simulink model "pos_pid_mbd_sl"  (Simulink 7.9)
settings: Solver=FixedStepDiscrete  StartTime=0.0  StopTime=tfinal  FixedStep=ts  RelTol=1e-3
values from neighbouring files (symbols this model uses):
  denpd = [1 -1.93941306281 0.939413062813]    [model_data.mat]
  dist = 0    [pos_pd_mbd.m]    (also in pos_pid2_mbd.m; pos_pid_mbd.m = 2; pos_pid_set.m; pos_tdof_mbd.m)
  Kd = -((p1+p2+p3)*T + 1)/K    [ipd_ff.m]    (also in pid_compare.m; pos_id_verify.m = 0; pos_pd_mbd.m = -((p1+p2)*T + 1)/K; pos_pid2_mbd.m)
  Ki = -p1*p2*p3*T/K    [ipd_ff.m]    (also in pid_compare.m; pos_id_verify.m = 0; pos_pd_mbd.m = 0; pos_pid2_mbd.m)
  Kp = (p1*p2 + p2*p3 + p3*p1)*T/K    [ipd_ff.m]    (also in pid_compare.m; pos_id_verify.m = Kp_id; pos_pd_mbd.m = p1*p2*T/K; pos_pid2_mbd.m)
  numpd = [0 0.223445736614 0.218838904848]    [model_data.mat]
  r = 60    [pos_id_step.m]    (also in pos_pd_mbd.m; pos_pid2_mbd.m; pos_pid_mbd.m; pos_pid_set.m)
  r_cyc = 8    [pos_id_step.m]    (also in pos_pd_mbd.m = 4; pos_pid2_mbd.m = 4; pos_pid_mbd.m = 4; pos_pid_set.m = 4)
  ts = 1/50    (= 0.02)    [sim_init.m]    (also in sim_param.mat)
undefined symbols (not defined in the file or in its folder): DiscIntNeverNeededParam
libraries: arduino_io_lib x5, simulink x2
settings Model: Creator=hirata  LastModifiedBy=hirata
settings DebuggingCC: FcnCallInpInsideContextMsg=Use local settings
settings GRTTargetCC: CombineOutputUpdateFcns=off  GRTInterface=on

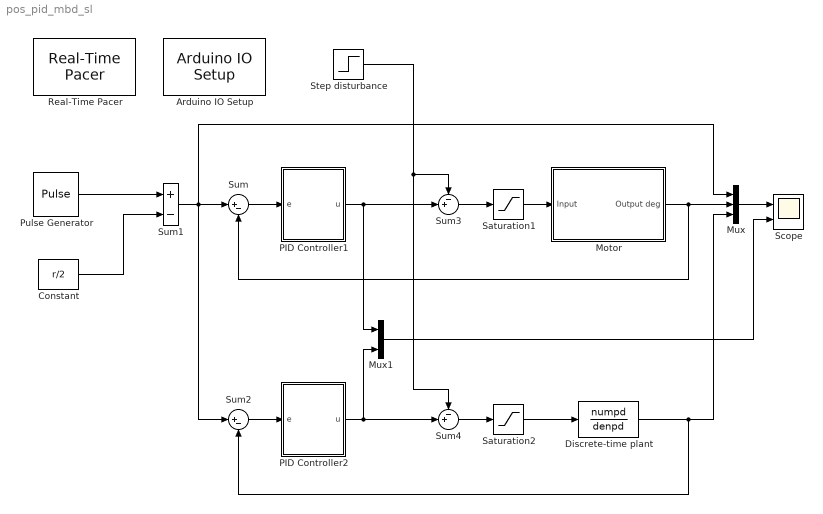
== system pos_pid_mbd_sl ==
  Arduino IO Setup : arduino_io_lib/Arduino IO Setup  Priority=3  arduinoVar=Temporary arduino variable: Arduino1  workspaceVarName=a  comPort=COM3
  Constant : Constant  Value=r/2
  Discrete-time plant : DiscreteTransferFcn  Numerator=numpd  Denominator=denpd
  Motor : Subsystem
  Mux : Mux  Inputs=3
  Mux1 : Mux  Inputs=2
  PID Controller1 : Subsystem
  PID Controller2 : Subsystem
  Pulse Generator : DiscretePulseGenerator  PulseType=Time based  Amplitude=r  Period=r_cyc  PulseWidth=50
  Real-Time Pacer : arduino_io_lib/Real-Time Pacer  simTimePerRealTime=1
  Saturation1 : Saturate  UpperLimit=5  LowerLimit=-5
  Saturation2 : Saturate  UpperLimit=5  LowerLimit=-5
  Scope : Scope  NumInputPorts=2
      settings: TimeRange=8  YMin=-80~-5  YMax=80~5  SaveName=yout
  Step disturbance : Step  Time=r_cyc/4  After=dist  SampleTime=ts
  Sum : Sum  Inputs=|+-
  Sum1 : Sum  Inputs=+-
  Sum2 : Sum  Inputs=|+-
  Sum3 : Sum  Inputs=-+|
  Sum4 : Sum  Inputs=-+|
  wires:
  PID Controller1/1(u) -> Mux1/1, Sum3/2
  Sum/1 -> PID Controller1/1(e)
  Sum1/1 -> Sum/1, Mux/1, Sum2/1
  Motor/1(Output deg) -> Sum/2, Mux/2
  Pulse Generator/1 -> Sum1/1
  Constant/1 -> Sum1/2
  Mux/1 -> Scope/1
  PID Controller2/1(u) -> Mux1/2, Sum4/2
  Sum2/1 -> PID Controller2/1(e)
  Mux1/1 -> Scope/2
  Discrete-time plant/1 -> Sum2/2, Mux/3
  Step disturbance/1 -> Sum4/1, Sum3/1
  Sum3/1 -> Saturation1/1
  Sum4/1 -> Saturation2/1
  Saturation1/1 -> Motor/1(Input)
  Saturation2/1 -> Discrete-time plant/1

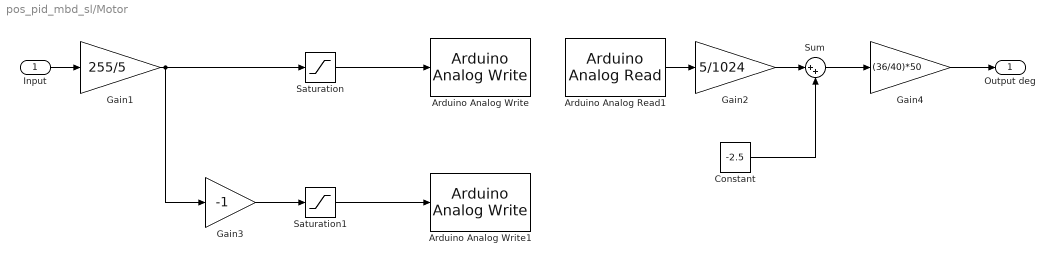
== system pos_pid_mbd_sl/Motor ==
  Input : Inport
  Arduino Analog Read1 : arduino_io_lib/Arduino Analog Read  arduinoVar=Temporary arduino variable: Arduino1  arduinoPin=0  T=ts
  Arduino Analog Write : arduino_io_lib/Arduino Analog Write  arduinoVar=Temporary arduino variable: Arduino1  arduinoPin=3  T=ts
  Arduino Analog Write1 : arduino_io_lib/Arduino Analog Write  arduinoVar=Temporary arduino variable: Arduino1  arduinoPin=5  T=ts
  Constant : Constant  Value=-2.5
  Gain1 : Gain  Gain=255/5
  Gain2 : Gain  Gain=5/1024
  Gain3 : Gain  Gain=-1
  Gain4 : Gain  Gain=(36/40)*50
  Saturation : Saturate  UpperLimit=255  LowerLimit=0
  Saturation1 : Saturate  UpperLimit=255  LowerLimit=0
  Sum : Sum  Inputs=|++
  Output deg : Outport
  wires:
  Input/1 -> Gain1/1
  Arduino Analog Read1/1 -> Gain2/1
  Saturation/1 -> Arduino Analog Write/1
  Gain1/1 -> Gain3/1, Saturation/1
  Saturation1/1 -> Arduino Analog Write1/1
  Gain4/1 -> Output deg/1
  Gain2/1 -> Sum/1
  Sum/1 -> Gain4/1
  Constant/1 -> Sum/2
  Gain3/1 -> Saturation1/1

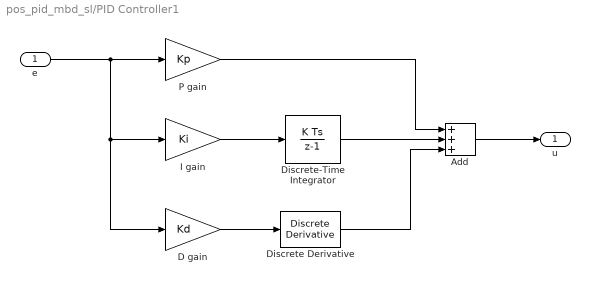
== system pos_pid_mbd_sl/PID Controller1 ==
  e : Inport
  Add : Sum  Inputs=+++
  D gain : Gain  Gain=Kd
  Discrete Derivative : simulink/Discrete/Discrete Derivative  gainval=1.0  ICPrevScaledInput=0.0  InputProcessing=Inherited  OutMin=[]  OutMax=[]  OutDataType=fixdt(1, 16)  OutScaling=2^-10  DoSatur=off
  Discrete-Time Integrator : DiscreteIntegrator  SampleTime=ts  ICPrevOutput=DiscIntNeverNeededParam  ICPrevScaledInput=DiscIntNeverNeededParam
  I gain : Gain  Gain=Ki
  P gain : Gain  Gain=Kp
  u : Outport
  wires:
  I gain/1 -> Discrete-Time Integrator/1
  P gain/1 -> Add/1
  Discrete-Time Integrator/1 -> Add/2
  e/1 -> P gain/1, I gain/1, D gain/1
  Add/1 -> u/1
  Discrete Derivative/1 -> Add/3
  D gain/1 -> Discrete Derivative/1

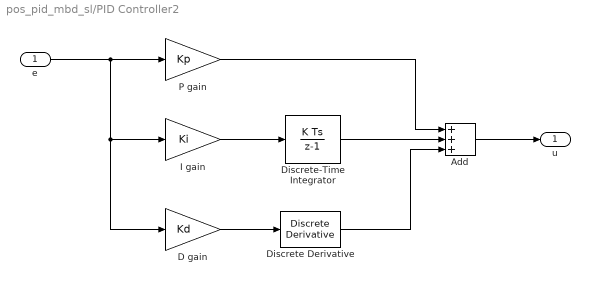
== system pos_pid_mbd_sl/PID Controller2 ==
  e : Inport
  Add : Sum  Inputs=+++
  D gain : Gain  Gain=Kd
  Discrete Derivative : simulink/Discrete/Discrete Derivative  gainval=1.0  ICPrevScaledInput=0.0  InputProcessing=Inherited  OutMin=[]  OutMax=[]  OutDataType=fixdt(1, 16)  OutScaling=2^-10  DoSatur=off
  Discrete-Time Integrator : DiscreteIntegrator  SampleTime=ts  ICPrevOutput=DiscIntNeverNeededParam  ICPrevScaledInput=DiscIntNeverNeededParam
  I gain : Gain  Gain=Ki
  P gain : Gain  Gain=Kp
  u : Outport
  wires:
  I gain/1 -> Discrete-Time Integrator/1
  P gain/1 -> Add/1
  Discrete-Time Integrator/1 -> Add/2
  e/1 -> P gain/1, I gain/1, D gain/1
  Add/1 -> u/1
  Discrete Derivative/1 -> Add/3
  D gain/1 -> Discrete Derivative/1
